simulink model "FMRadioReceiver"  (R2017b)
settings: Solver=FixedStepDiscrete  StartTime=0.0  StopTime=inf  RelTol=1e-3
PreLoadFcn:
  | stereoFMRxParams = getParamsFMExamplesAD9361AD9364;
InitFcn:
  | stereoFMRxParams = getParamsFMExamplesAD9361AD9364;
undefined symbols (not defined in the file or in its folder): F
libraries: adirfsom_lib x1, simulink x1, dspsnks4 x1, commanabbnd3 x1
CloseFcn:
  | clear stereoFMRxParams
Description:
  | This model uses Zynq-based SDR hardware with Analog Devices(TM) FMCOMMS2, FMCOMMS3 or FMCOMMS4 to perform FM stereo demodulation using Simulink(R).
settings Model: SimulationMode=accelerator  Creator=The MathWorks, Inc.  LastModifiedBy=ppradhan
settings DataIOCC: SaveFormat=Structure  SaveOutput=off  SignalLogging=off  DSMLogging=off  SaveTime=off
settings OptimizationCC: ExpressionDepthLimit=2147483647  EfficientMapNaN2IntZero=off  LifeSpan=inf  SimCompilerOptimization=on
settings DebuggingCC: UnderspecifiedInitializationDetection=Classic  MergeDetectMultiDrivingBlocksExec=none  SolverPrmCheckMsg=warning  InheritedTsInSrcMsg=none  MultiTaskCondExecSysMsg=none  ParameterPrecisionLossMsg=none  FcnCallInpInsideContextMsg=warning  AllowSymbolicDim=off  StateNameClashWarn=warning  SFUnexpectedBacktrackingDiag=warning  SFNoUnconditionalDefaultTransitionDiag=warning  SFExecutionAtInitializationDiag=none
settings HardwareCC: ProdBitPerPointer=32  ProdBitPerSizeT=32  ProdBitPerPtrDiffT=32  ProdLargestAtomicFloat=None  ProdIntDivRoundTo=Undefined  ProdEndianess=Unspecified  ProdWordSize=32  ProdHWDeviceType=32-bit Generic  TargetBitPerPointer=64  TargetBitPerSizeT=64  TargetBitPerPtrDiffT=64  TargetLongLongMode=on  TargetIntDivRoundTo=Zero  TargetEndianess=LittleEndian  TargetWordSize=64  TargetHWDeviceType=Generic->MATLAB Host Computer  ProdEqTarget=off
settings ModelReferenceCC: PropagateSignalLabelsOutOfModel=off
settings SFSimCC: SimIntegrity=off
settings RTWCC: CustomSourceCode=|
  | #include <stdio.h>
  | #include <stdlib.h>
settings CodeAppCC: MaxIdLength=128  StateflowObjectComments=on
settings GRTTargetCC: TargetLangStandard=C89/C90 (ANSI)  GeneratePreprocessorConditionals=Disable all  CombineOutputUpdateFcns=off  GRTInterface=on
settings ConfigComp: CovMetricSettings=dw  CovHtmlReporting=on  CovSaveCumulativeToWorkspaceVar=on  CovSaveSingleToWorkspaceVar=on  CovExternalEMLEnable=off  CovSFcnEnable=off

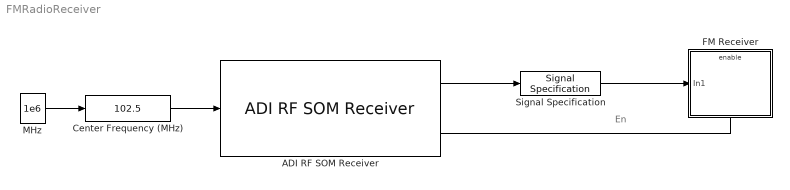
== system FMRadioReceiver ==
  note: En
  ADI RF SOM Receiver : adirfsom_lib/ADI RF SOM Receiver  IPAddress=192.168.3.2  CenterFrequencySource=Input port  CenterFrequency=2400000000  GainSource=AGC Fast Attack  Gain=1  ChannelMapping=1  BasebandSampleRate=stereoFMRxParams.RadioSampleRate  EnableBurstMode=off  NumFramesInBurst=20  OutputDataType=single  SamplesPerFrame=stereoFMRxParams.RadioFrameLength  LostSamplesOutputPort=off  RSSIOutputPort=off  DMATimeoutValue=1  blockMode=Normal  SimulateUsing=Code generation  EnableQuadratureTracking=on  EnableRFDCTracking=on  EnableBasebandDCTracking=on  BypassUserLogic=on  ShowAdvancedProperties=on  ShowInternalProperties=off  subDeviceList=zynqReceiver  sdrExecutionMode=HW  dataUDPPort=-1  ctrlUDPPort=-1  SourceSelect=RF data  SourceConfiguration1=1023  FIRCoefficientSize=[ 128; 128 ]  FIRCoefficients=[ 55, -54, 42, -126, -123, -317, -399, -581, -646, -711, -634, -507, -263, -10, 255, 424, 492, 401, 201, -84, -352, -540, -566, -423, -126, 234, 562, 738, 701, 429, -5, -490, -866, -1007, -834, -372, 266, 891, 1301, 1334, 936, 178, -733, -1524, -1917, -1731, -944, 274, 1590, 2585, 2881, 2255, 741, -1344, -3435, -4850, -4942, -3285, 197, 5169, 10923, 16509, 20932, 23375, 23375, 20932, 16509, 10923, 5169, 197, -3285, -4942, -4850, -3435, -1344, 741, 2255, 2881, 2585, 1590, 274, -944, -1731, -1917, -1524, -733, 178, 936, 1334, 1301, 891, 266, -372, -834, -1007, -866, -490, -5, 429, 701, 738, 562, 234, -126, -423, -566, -540, -352, -84, 201, 401, 492, 424, 255, -10, -263, -507, -634, -711, -646, -581, -399, -317, -123, -126, 42, -54, 55; 190, -88, 329, -40, 239, -99, -24, -349, -377, -611, -573, -604, -395, -229, 66, 239, 394, 350, 227, -46, -300, -534, -593, -506, -221, 137, 512, 737, 765, 526, 103, -420, -852, -1069, -947, -512, 156, 841, 1341, 1450, 1100, 333, -638, -1531, -2028, -1922, -1152, 115, 1544, 2677, 3099, 2535, 997, -1205, -3479, -5095, -5345, -3750, -199, 4965, 11002, 16895, 21580, 24172, 24172, 21580, 16895, 11002, 4965, -199, -3750, -5345, -5095, -3479, -1205, 997, 2535, 3099, 2677, 1544, 115, -1152, -1922, -2028, -1531, -638, 333, 1100, 1450, 1341, 841, 156, -512, -947, -1069, -852, -420, 103, 526, 765, 737, 512, 137, -221, -506, -593, -534, -300, -46, 227, 350, 394, 239, 66, -229, -395, -604, -573, -611, -377, -349, -24, -99, 239, -40, 329, -88, 190 ]  FIRGain=[ 0; -12 ]  FIRDecimInterpFactor=[ 4; 4 ]  AnalogFilterCutoff=[ 3152524; 3161715 ]  FilterPathRates=[ 983040000, 122880000, 61440000, 30720000, 15360000, 3840000; 983040000, 122880000, 61440000, 30720000, 15360000, 3840000 ]  FilterDesignTypeForTx=DefaultFilterFromOther  FilterDesignTypeForRx=DefaultFilter  BISTLoopbackConfig=No Loopback  BISTPRBSMode=PRBS Disable  BISTToneMode=Tone Disable  BISTToneFrequency=F/32  BISTToneLevel=-6  BISTChannelMask=0  DataIsComplex=on
      settings: SourceProductName=Communications System Toolbox Support Package for Xilinx Zynq-Based Radio
  Center Frequency (MHz) : simulink/Math Operations/Slider Gain  gain=102.5  low=87.5  high=1002.5
  FM Receiver : Subsystem  TreatAsAtomicUnit=on
      mask Display:
      | plot(0,0,100,100,[5+4.5*[0:.15:10] 50 50 50 50+4.5*[0:10]],[85+10*[sin([0:.15:10]*pi*2+cumsum(sin([0:.15:10]*pi/5))/2)] 85 99 75   10*sin([0:10]*pi/5)+85])
      | disp('\nFM\nBroadcast\nDemodulator')
  MHz : Constant  Value=1e6  VectorParams1D=off  SampleTime=stereoFMRxParams.RadioFrameLength/stereoFMRxParams.RadioSampleRate  FramePeriod=-1
  Signal Specification : SignalSpecification  SampleTime=stereoFMRxParams.RadioFrameLength/stereoFMRxParams.RadioSampleRate
  wires:
  ADI RF SOM Receiver/2 -> FM Receiver/Enable
  MHz/1 -> Center Frequency (MHz)/1
  Center Frequency (MHz)/1 -> ADI RF SOM Receiver/1
  ADI RF SOM Receiver/1 -> Signal Specification/1
  Signal Specification/1 -> FM Receiver/1(In1)

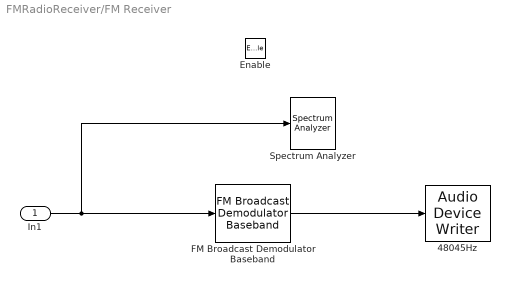
== system FMRadioReceiver/FM Receiver ==
  In1 : Inport
  Enable : EnablePort
  48045Hz : dspsnks4/Audio Device Writer  Driver=DirectSound  Device=Default  InheritSampleRate=on  SampleRate=44100  BitDepth=16-bit integer  BufferSize=4096  NumBuffers=10  DefaultOutputChannelMapping=on  OutputChannelMapping=1:2  OutputNumUnderrunSamples=off  DriverIdx=1  DeviceWarnFlag=''
  FM Broadcast Demodulator Baseband : commanabbnd3/FM Broadcast Demodulator Baseband  SampleRate=stereoFMRxParams.RadioSampleRate  FrequencyDeviation=stereoFMRxParams.FrequencyDeviation  FilterTimeConstant=stereoFMRxParams.FilterTimeConstant  AudioSampleRate=stereoFMRxParams.AudioSampleRate  PlaySound=off  BufferSize=stereoFMRxParams.BufferSize  Stereo=off  SimulateUsing=Code generation
      settings: SourceProductName=Communications System Toolbox  SourceProductBaseCode=CM
  Spectrum Analyzer : SpectrumAnalyzer
  wires:
  In1/1 -> Spectrum Analyzer/1, FM Broadcast Demodulator Baseband/1
  FM Broadcast Demodulator Baseband/1 -> 48045Hz/1
